simulink model "SimpleMath"  (R2023a)
settings: Solver=FixedStepDiscrete  StartTime=0.0  StopTime=10.0  FixedStep=0.01  RelTol=1e-3
model workspace (MAT data in the model file):
  In1 = MoTeC.InParameter
  In1.M1Name = 'In1'
  In1.DataType = 'single'
  In1.Complexity = 'real'
  In1.Dimensions = [0 0]
  In2 = MoTeC.InParameter
  In2.M1Name = 'In2'
  In2.DataType = 'single'
  In2.Complexity = 'real'
  In2.Dimensions = [0 0]
  Out1 = MoTeC.Channel
  Out1.M1Name = 'Out1'
  Out1.DataType = 'single'
  Out1.Dimensions = -1
  Out1.DimensionsMode = 'auto'
  Out1.Complexity = 'auto'
  Out1.SampleTime = -1
  Out1.SamplingMode = 'auto'
settings Model: Creator=Raheel Farouk  LastModifiedBy=Raheel Farouk
settings OptimizationCC: DefaultParameterBehavior=Inlined  EnhancedBackFolding=on  PassReuseOutputArgsAs=Individual arguments  ZeroExternalMemoryAtStartup=off  ZeroInternalMemoryAtStartup=off  InitFltsAndDblsToZero=on  MaxStackSize=2048  OptimizeBlockOrder=speed  DifferentSizesBufferReuse=on  OptimizationCustomize=off  EfficientTunableParamExpr=on
settings DebuggingCC: ParameterTunabilityLossMsg=error
settings HardwareCC: ProdBitPerPointer=32  ProdBitPerSizeT=32  ProdBitPerPtrDiffT=32  ProdLargestAtomicInteger=Long  ProdLargestAtomicFloat=Double  ProdEndianess=BigEndian  ProdWordSize=32  ProdHWDeviceType=Freescale->32-bit PowerPC
settings ModelReferenceCC: UpdateModelReferenceTargets=Force
settings SFSimCC: MATLABDynamicMemAlloc=off
settings RTWCC: Description=Create MoTeC M1 Package  SystemTargetFile=MoTeC.tlc  TemplateMakefile=MoTeCUserlibMakefile.tmf  PostCodeGenCommand=MoTeCUtil.m1_post_process(buildInfo)
settings CodeAppCC: ForceParamTrailComments=on  IgnoreCustomStorageClasses=off  OperatorAnnotations=on  SimulinkDataObjDesc=on  SFDataObjDesc=on  InsertBlockDesc=on
settings STFCustomTargetCC: MultiwordLength=256  GenerateSampleERTMain=on  ConcurrentExecutionCompliant=off  CombineOutputUpdateFcns=on  ERTCustomFileBanners=on  SupportContinuousTime=off  SupportNonInlinedSFcns=off  RemoveResetFunc=on  MATLABClassNameForMDSCustomization=Simulink.SoftwareTarget.ERTCustomization  GRTInterface=off  UseToolchainInfoCompliant=off  SystemTargetFile=MoTeC.tlc
settings ERTTargetCC: TargetLangStandard=C99 (ISO)  GenerateSampleERTMain=on  ParMdlRefBuildCompliant=off  CompOptLevelCompliant=off  ConcurrentExecutionCompliant=off  ModelStepFunctionPrototypeControlCompliant=off  CPPClassGenCompliant=off  UseToolchainInfoCompliant=off  InlinedParameterPlacement=NonHierarchical  ERTCustomFileTemplate=MoTeCFileProcess.tlc  EnableUserReplacementTypes=on

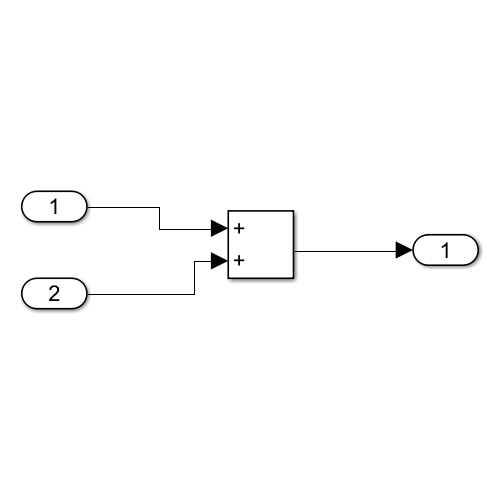
[thumbnail: Simulink's stored preview of the top-level diagram]
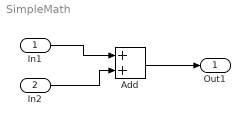
== system SimpleMath ==
  In1 : Inport
  In2 : Inport  Port=2
  Add : Sum
  Out1 : Outport
  wires:
  In1/1 -> Add/1
  In2/1 -> Add/2
  Add/1 -> Out1/1
